simulink model "with_sssc"  (Simulink 7.3)
settings: Solver=FixedStepDiscrete  SolverMode=SingleTasking  StartTime=0.0  StopTime=0.8  FixedStep=Ts  RelTol=1e-3
PreLoadFcn:
  | Ts=1/512/60;
undefined symbols (not defined in the file): DiscIntNeverNeededParam
libraries: powerlib x54, powerlib_extras x38, simulink_extras x2, simulink x1
(part 3 of 7)

== system with_sssc/sssc Controller/SH Control (STATCOM)/DC Balance Regulator ==
  Iq_avg : Inport  PortDimensions=1  OutDataType=sfix(16)  OutScaling=2^0
  +/-Vdc/2 : Inport  Port=2  PortDimensions=2  OutDataType=sfix(16)  OutScaling=2^0
  " Mean value" : Subsystem  mask(Discrete Mean value){Freq=60, Vinit=0, Ts=Ts}
      mask prompts: Freq "Fundamental frequency (Hz):"; Vinit "Initial input (DC component):"; Ts "Sample time:"
      mask help:
      | This block computes the mean value of the input signal over a running window of one cycle of the specified fundamental frequency.
      | For the first cycle of simulation, the output is held constant to the value specified by the parameter "Initial input".
      mask init:
      | SamplesPerCycle=1/Freq/Ts;
      | RoundSamplesPerCycle=round(SamplesPerCycle);
      | Delay=RoundSamplesPerCycle*Ts - Ts/2;
      | Correction=SamplesPerCycle/RoundSamplesPerCycle - 1;
  Abs : Abs  OutDataType=sfix(16)  OutScaling=2^0  SaturateOnIntegerOverflow=on
  D_Alpha(Manual) : Constant  Value=0  OutDataType=sfix(16)  OutScaling=2^0
  D_Alpha1 : Constant  Value=0  OutDataType=sfix(16)  OutScaling=2^0
  D_Alpha2 : Constant  Value=0  OutDataType=sfix(16)  OutScaling=2^0
  D_Alpha5 : Constant  Value=0.1  OutDataType=sfix(16)  OutScaling=2^0
  Demux : Demux  Outputs=2
  Gain : Gain  Gain=0  ParameterDataType=sfix(16)  ParameterScaling=2^0  OutDataType=sfix(16)  OutScaling=2^0  SaturateOnIntegerOverflow=on  OutDataTypeStr=Inherit: Same as input  ParamDataTypeStr=Inherit: Same as input
  Gain1 : Gain  Gain=-1  ParameterDataType=sfix(16)  ParameterScaling=2^0  OutDataType=sfix(16)  OutScaling=2^0  SaturateOnIntegerOverflow=on  OutDataTypeStr=Inherit: Same as input  ParamDataTypeStr=Inherit: Same as input
  Mode : Constant  OutDataType=sfix(16)  OutScaling=2^0
  Multiport Switch : MultiPortSwitch  OutDataType=sfix(16)  OutScaling=2^0  SaturateOnIntegerOverflow=on  InputSameDT=on
  PI Regulator : Subsystem  mask(Discrete PI Controller){Kp=0.001, Ki=0.01, Par_Limits=[2 -2], Init=0, Ts=Ts}
      mask prompts: Kp "Proportional gain (Kp):"; Ki "Integral gain (Ki):"; Par_Limits "Output limits: [ Upper   Lower ]"; Init "Output initial value:"; Ts "Sample time:"
      mask help: This block implements a discrete PI controller.
      mask init:
      | UpperLimit=Par_Limits(1);
      | LowerLimit=Par_Limits(2);
      mask Display: disp('PI');
  Relational Operator : RelationalOperator  Operator=<=  InputSameDT=on
  Relational Operator1 : RelationalOperator  Operator=<  InputSameDT=on
  Sum2 : Sum  Inputs=-+  OutDataType=sfix(16)  OutScaling=2^0  SaturateOnIntegerOverflow=on  InputSameDT=on  OutDataTypeStr=Inherit: Same as first input
  Switch : Switch  Threshold=0.5  OutDataType=sfix(16)  OutScaling=2^0  SaturateOnIntegerOverflow=on  InputSameDT=on
  Switch1 : Switch  Threshold=0.5  OutDataType=sfix(16)  OutScaling=2^0  SaturateOnIntegerOverflow=on  InputSameDT=on
  D_Alpha : Outport  OutDataType=sfix(16)  OutScaling=2^0
  wires:
  Demux/2 -> Sum2/2
  Demux/1 -> Sum2/1
  +/-Vdc/2/1 -> Demux/1
  Iq_avg/1 -> Relational Operator/1, Abs/1
  Sum2/1 -> " Mean value"/1(In)
  Switch1/1 -> PI Regulator/1(Error)
  Gain/1 -> Switch1/1
  " Mean value"/1(Mean) -> Gain/1, Switch1/3
  D_Alpha1/1 -> Relational Operator/2
  Abs/1 -> Relational Operator1/1
  D_Alpha5/1 -> Relational Operator1/2
  Gain1/1 -> Switch/3
  Relational Operator/1 -> Switch/2
  Switch/1 -> Multiport Switch/2  "Auto"
  D_Alpha2/1 -> Multiport Switch/4  "Off"
  Mode/1 -> Multiport Switch/1
  PI Regulator/1(Out) -> Switch/1, Gain1/1
  D_Alpha(Manual)/1 -> Multiport Switch/3  "Man"
  Multiport Switch/1 -> D_Alpha/1
  Relational Operator1/1 -> Switch1/2, PI Regulator/2(Reset)

== system with_sssc/sssc Controller/SH Control (STATCOM)/Firing Pulses Generator ==
  Alpha : Inport  PortDimensions=1  OutDataType=sfix(16)  OutScaling=2^0
  Sigma : Inport  Port=2  PortDimensions=1  OutDataType=sfix(16)  OutScaling=2^0
  wt : Inport  Port=3  PortDimensions=1  OutDataType=sfix(16)  OutScaling=2^0
  D_Alpha : Inport  Port=4  PortDimensions=1  OutDataType=sfix(16)  OutScaling=2^0
  " Deg->Rad" : Gain  Gain=pi/180  ParameterDataType=sfix(16)  ParameterScaling=2^0  OutDataType=sfix(16)  OutScaling=2^0  SaturateOnIntegerOverflow=on  OutDataTypeStr=Inherit: Same as input  ParamDataTypeStr=Inherit: Same as input
  Bridge 1D : Subsystem
  "Bridge 1Y " : Subsystem
  Bridge 2D : Subsystem
  Bridge 2Y : Subsystem
  Constant : Constant  Value=[0 -30 -15 -45]*pi/180 + 7.5*pi/180  OutDataType=sfix(16)  OutScaling=2^0
  Deg->Rad : Gain  Gain=pi/180  ParameterDataType=sfix(16)  ParameterScaling=2^0  OutDataType=sfix(16)  OutScaling=2^0  SaturateOnIntegerOverflow=on  OutDataTypeStr=Inherit: Same as input  ParamDataTypeStr=Inherit: Same as input
  "Deg->Rad " : Gain  Gain=pi/180  ParameterDataType=sfix(16)  ParameterScaling=2^0  OutDataType=sfix(16)  OutScaling=2^0  SaturateOnIntegerOverflow=on  OutDataTypeStr=Inherit: Same as input  ParamDataTypeStr=Inherit: Same as input
  Demux : Demux
  Mux : Mux  Inputs=[12 12 12 12]
  Sum : Sum  OutDataType=sfix(16)  OutScaling=2^0  SaturateOnIntegerOverflow=on  InputSameDT=on  OutDataTypeStr=Inherit: Same as first input
  Pulses : Outport  OutDataType=sfix(16)  OutScaling=2^0
  wires:
  Alpha/1 -> Deg->Rad/1
  Constant/1 -> Sum/2
  Sum/1 -> Demux/1
  "Bridge 1Y "/1(Pulses) -> Mux/1
  Mux/1 -> Pulses/1
  Demux/1 -> "Bridge 1Y "/1(wt)
  Sigma/1 -> "Deg->Rad "/1
  Demux/2 -> Bridge 1D/1(wt)
  Demux/3 -> Bridge 2Y/1(wt)
  Demux/4 -> Bridge 2D/1(wt)
  Deg->Rad/1 -> "Bridge 1Y "/2(Alpha), Bridge 1D/2(Alpha), Bridge 2Y/2(Alpha), Bridge 2D/2(Alpha)
  "Deg->Rad "/1 -> "Bridge 1Y "/3(Sigma), Bridge 1D/3(Sigma), Bridge 2Y/3(Sigma), Bridge 2D/3(Sigma)
  " Deg->Rad"/1 -> Bridge 2D/4(D_Alpha), Bridge 2Y/4(D_Alpha), Bridge 1D/4(D_Alpha), "Bridge 1Y "/4(D_Alpha)
  D_Alpha/1 -> " Deg->Rad"/1
  Bridge 1D/1(Pulses) -> Mux/2
  Bridge 2Y/1(Pulses) -> Mux/3
  Bridge 2D/1(Pulses) -> Mux/4
  wt/1 -> Sum/1

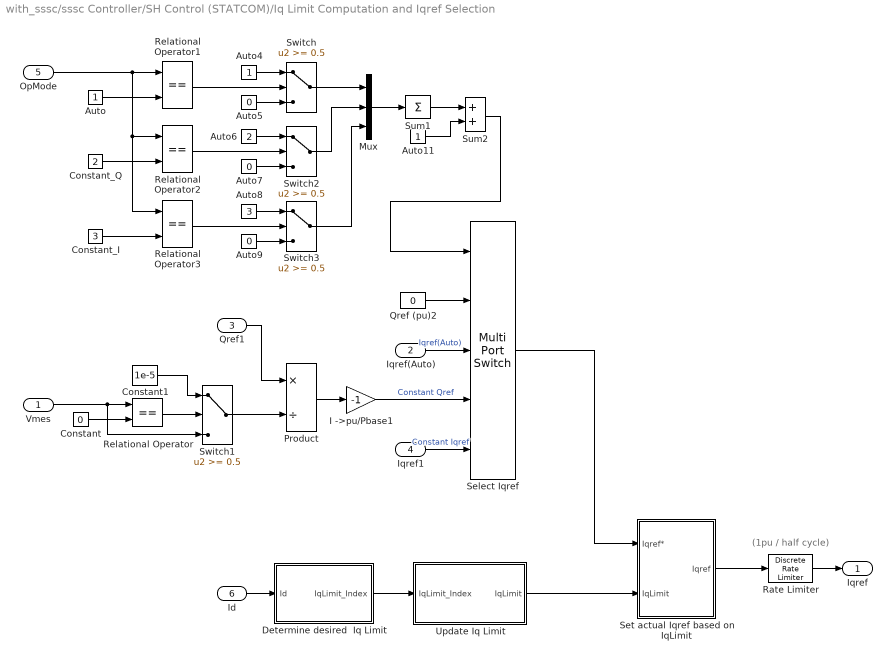
== system with_sssc/sssc Controller/SH Control (STATCOM)/Iq Limit Computation and Iqref Selection ==
  note: (1pu / half cycle)
  Vmes : Inport  OutDataType=sfix(16)  OutScaling=2^0
  Iqref(Auto) : Inport  Port=2  OutDataType=sfix(16)  OutScaling=2^0
  Qref1 : Inport  Port=3  OutDataType=sfix(16)  OutScaling=2^0
  Iqref1 : Inport  Port=4  OutDataType=sfix(16)  OutScaling=2^0
  OpMode : Inport  Port=5  OutDataType=sfix(16)  OutScaling=2^0
  Id : Inport  Port=6  OutDataType=sfix(16)  OutScaling=2^0
  Auto : Constant  OutDataType=sfix(16)  OutScaling=2^0
  Auto11 : Constant  OutDataType=sfix(16)  OutScaling=2^0
  Auto4 : Constant  OutDataType=sfix(16)  OutScaling=2^0
  Auto5 : Constant  Value=0  OutDataType=sfix(16)  OutScaling=2^0
  Auto6 : Constant  Value=2  OutDataType=sfix(16)  OutScaling=2^0
  Auto7 : Constant  Value=0  OutDataType=sfix(16)  OutScaling=2^0
  Auto8 : Constant  Value=3  OutDataType=sfix(16)  OutScaling=2^0
  Auto9 : Constant  Value=0  OutDataType=sfix(16)  OutScaling=2^0
  Constant : Constant  Value=0  OutDataType=sfix(16)  OutScaling=2^0
  Constant1 : Constant  Value=1e-5  OutDataType=sfix(16)  OutScaling=2^0
  Constant_I : Constant  Value=3  OutDataType=sfix(16)  OutScaling=2^0
  Constant_Q : Constant  Value=2  OutDataType=sfix(16)  OutScaling=2^0
  Determine desired  Iq Limit : Subsystem
  I ->pu/Pbase1 : Gain  Gain=-1  ParameterDataType=sfix(16)  ParameterScaling=2^0  OutDataType=sfix(16)  OutScaling=2^0  SaturateOnIntegerOverflow=on  OutDataTypeStr=Inherit: Same as input  ParamDataTypeStr=Inherit: Same as input
  Mux : Mux  Inputs=3
  Product : Product  Inputs=*/  OutDataType=sfix(16)  OutScaling=2^0  SaturateOnIntegerOverflow=on  InputSameDT=on  OutDataTypeStr=Inherit: Same as first input
  Qref (pu)2 : Constant  Value=0  OutDataType=sfix(16)  OutScaling=2^0
  "Rate Limiter " : powerlib_extras/Discrete  Control Blocks/Discrete Rate Limiter  DialogController=POWERSYS.PowerSysDialog  SystemSampleTime=-1  R=120  F=-120  Vinit=-0.33  Ts=Ts
  Relational Operator{,1..3} (4 alike) : RelationalOperator  Operator===  InputSameDT=on
  Select Iqref : MultiPortSwitch  Inputs=4  OutDataType=sfix(16)  OutScaling=2^0  SaturateOnIntegerOverflow=on  InputSameDT=on
  Set actual Iqref based on IqLimit : Subsystem
  Sum1 : Sum  Inputs=1  OutDataType=sfix(16)  OutScaling=2^0  SaturateOnIntegerOverflow=on  InputSameDT=on  OutDataTypeStr=Inherit: Same as first input
  Sum2 : Sum  OutDataType=sfix(16)  OutScaling=2^0  SaturateOnIntegerOverflow=on  InputSameDT=on  OutDataTypeStr=Inherit: Same as first input
  Switch{,1..3} (4 alike) : Switch  Threshold=0.5  OutDataType=sfix(16)  OutScaling=2^0  SaturateOnIntegerOverflow=on  InputSameDT=on
  Update Iq Limit : Subsystem
  Iqref : Outport  OutDataType=sfix(16)  OutScaling=2^0
  wires:
  Switch2/1 -> Mux/2
  Auto11/1 -> Sum2/2
  Sum1/1 -> Sum2/1
  Switch3/1 -> Mux/3
  Mux/1 -> Sum1/1
  Switch/1 -> Mux/1
  Auto9/1 -> Switch3/3
  Auto8/1 -> Switch3/1
  Relational Operator3/1 -> Switch3/2
  Auto7/1 -> Switch2/3
  Auto6/1 -> Switch2/1
  Relational Operator2/1 -> Switch2/2
  Auto5/1 -> Switch/3
  Auto4/1 -> Switch/1
  Relational Operator1/1 -> Switch/2
  OpMode/1 -> Relational Operator3/1, Relational Operator2/1, Relational Operator1/1
  Constant_I/1 -> Relational Operator3/2
  Constant_Q/1 -> Relational Operator2/2
  Auto/1 -> Relational Operator1/2
  Sum2/1 -> Select Iqref/1
  Vmes/1 -> Relational Operator/1, Switch1/3
  Qref1/1 -> Product/1
  Relational Operator/1 -> Switch1/2
  Constant1/1 -> Switch1/1
  Switch1/1 -> Product/2
  Constant/1 -> Relational Operator/2
  Product/1 -> I ->pu/Pbase1/1
  Iqref1/1 -> Select Iqref/5  "Constant Iqref"
  Iqref(Auto)/1 -> Select Iqref/3  "Iqref(Auto)"
  I ->pu/Pbase1/1 -> Select Iqref/4  "Constant Qref"
  Qref (pu)2/1 -> Select Iqref/2
  Select Iqref/1 -> Set actual Iqref based on IqLimit/1(Iqref*)
  Determine desired  Iq Limit/1(IqLimit_Index) -> Update Iq Limit/1(IqLimit_Index)
  Update Iq Limit/1(IqLimit) -> Set actual Iqref based on IqLimit/2(IqLimit)
  Set actual Iqref based on IqLimit/1(Iqref) -> "Rate Limiter "/1
  "Rate Limiter "/1 -> Iqref/1
  Id/1 -> Determine desired  Iq Limit/1(Id)

== system with_sssc/sssc Controller/SH Control (STATCOM)/Measurement System ==
  Vabc : Inport  PortDimensions=3  OutDataType=sfix(16)  OutScaling=2^0
  Iabc : Inport  Port=2  PortDimensions=3  OutDataType=sfix(16)  OutScaling=2^0
  Freq : Inport  Port=3  PortDimensions=1  OutDataType=sfix(16)  OutScaling=2^0
  wt : Inport  Port=4  PortDimensions=1  OutDataType=sfix(16)  OutScaling=2^0
  Discrete Variable Frequency Mean value : powerlib_extras/Discrete Measurements/Discrete Variable Frequency Mean value  DialogController=POWERSYS.PowerSysDialog  SystemSampleTime=-1  Finit=60  Fmin=45  Vinit=0  Ts=Ts
  Discrete  2nd-Order Filter : powerlib_extras/Discrete  Control Blocks/Discrete  2nd-Order Filter  DialogController=POWERSYS.PowerSysDialog  SystemSampleTime=-1  FilterType=Lowpass  Fo=1200  Zeta=0.707  Ts=Ts  Initialize=off  Vac_Init=[0.8 -25 60]  Vdc_Init=-0.4  PlotResponse=off  param1=[1 500 1]
  Discrete  2nd-Order Filter1 : powerlib_extras/Discrete  Control Blocks/Discrete  2nd-Order Filter  DialogController=POWERSYS.PowerSysDialog  SystemSampleTime=-1  FilterType=Lowpass  Fo=1200  Zeta=0.707  Ts=Ts  Initialize=off  Vac_Init=[0.8 -25 60]  Vdc_Init=-0.4  PlotResponse=off  param1=[1 500 1]
  Mux : Mux  Inputs=2
  PQ  Computaion : Subsystem
  Selector : Selector  InputPortWidth=2  IndexOptions=Index vector (dialog)  Indices=2  OutputSizes=1
  Selector1 : Selector  InputPortWidth=2  IndexOptions=Index vector (dialog)  Indices=1  OutputSizes=1
  Selector2 : Selector  InputPortWidth=3  IndexOptions=Index vector (dialog)  Indices=1:2  OutputSizes=1
  Trigonometric Function : Trigonometry
  Trigonometric Function1 : Trigonometry  Operator=cos
  Voltage measurement (Positive sequence) : Subsystem  mask(Discrete 3-phase PLL-Driven Positive-Sequence Fundamental Value){Finit=60, Par_Init=[1 0], Ts=Ts}
      mask prompts: Finit "Initial fundamental frequency (Hz):"; Par_Init "Initial input (positive component): [ Mag  Phase-relative-to-PLL(degrees) ]"; Ts "Sample time:"
      mask help:
      | For a supplied fundamental frequency (port Freq), this discrete block computes  the positive-sequence component (Magnitude and Phase)  of a set of three balanced or unbalanced signals (port abc) which may contain harmonics.
      |  Input port "Sin_Cos" (a two-dimension signal) provides the reference frame required for the computation..
      |  First and second outputs return respectively the magnitude and phase (in degrees relative to the PLL phase)) of the fundamental.
      | For the first cycle of simulation, the outputs are held constant to the values specified by the parameter "Initial input".
      mask init:
      | Real_Init=Par_Init(1)*cos(pi/180*Par_Init(2));
      | Imag_Init=Par_Init(1)*sin(pi/180*Par_Init(2));
  abc_to_dq0 Transformation : powerlib_extras/Measurements/abc_to_dq0 Transformation  DialogController=POWERSYS.PowerSysDialog  SystemSampleTime=-1
  Vmes : Outport  OutDataType=sfix(16)  OutScaling=2^0
  PQ : Outport  Port=2  OutDataType=sfix(16)  OutScaling=2^0
  Iq : Outport  Port=3  OutDataType=sfix(16)  OutScaling=2^0
  Iq_avg : Outport  Port=4  OutDataType=sfix(16)  OutScaling=2^0
  Id : Outport  Port=5  OutDataType=sfix(16)  OutScaling=2^0
  wires:
  Discrete  2nd-Order Filter/1 -> Id/1
  Selector1/1 -> Discrete  2nd-Order Filter/1
  Discrete Variable Frequency Mean value/1 -> Iq_avg/1
  Selector/1 -> Discrete  2nd-Order Filter1/1, Discrete Variable Frequency Mean value/2
  Freq/1 -> PQ  Computaion/3(Freq), Discrete Variable Frequency Mean value/1, Voltage measurement (Positive sequence)/2(Freq)
  abc_to_dq0 Transformation/1 -> Selector2/1
  PQ  Computaion/1(PQ(pu)) -> PQ/1
  Mux/1 -> Voltage measurement (Positive sequence)/3(Sin_Cos), abc_to_dq0 Transformation/2
  wt/1 -> Trigonometric Function1/1, Trigonometric Function/1
  Trigonometric Function1/1 -> Mux/2
  Trigonometric Function/1 -> Mux/1
  Vabc/1 -> Voltage measurement (Positive sequence)/1(abc)
  Voltage measurement (Positive sequence)/1(Mag) -> Vmes/1  "Vmes"
  Voltage measurement (Positive sequence)/2(VdVq) -> PQ  Computaion/1(Vd_Vq)
  Discrete  2nd-Order Filter1/1 -> Iq/1
  Iabc/1 -> abc_to_dq0 Transformation/1
  Selector2/1 -> Selector1/1, Selector/1, PQ  Computaion/2(Id_Iq)

== system with_sssc/sssc Controller/SH Control (STATCOM)/PLL ==
  note: Pierre Giroux, Gilbert Sybille
      | Power System Laboratory, IREQ
      | Hydro-Quebec
  note: Discrete 3-phase PLL
  Vabc (pu) : Inport  PortDimensions=3  OutDataType=sfix(16)  OutScaling=2^0
  Constant4 : Constant  Value=2*pi  OutDataType=sfix(16)  OutScaling=2^0
  Correction for delay : Gain  Gain=Nstep*Ts*2*pi  ParameterDataType=sfix(16)  ParameterScaling=2^0  OutDataType=sfix(16)  OutScaling=2^0  SaturateOnIntegerOverflow=on  OutDataTypeStr=Inherit: Same as input  ParamDataTypeStr=Inherit: Same as input
  Discrete PI Controller : powerlib_extras/Discrete  Control Blocks/Discrete PI Controller  DialogController=POWERSYS.PowerSysDialog  SystemSampleTime=-1  Kp=Kp  Ki=Ki  Par_Limits=2*pi*Finit*[1.25 0.75]  Init=2*pi*Finit  Ts=Ts
  Discrete Rate Limiter : powerlib_extras/Discrete  Control Blocks/Discrete Rate Limiter  DialogController=POWERSYS.PowerSysDialog  SystemSampleTime=-1  R=10  F=-10  Vinit=Finit  Ts=Ts
  Discrete Variable Frequency Mean value : Subsystem  mask(Discrete Variable-Frequency Mean Value){Finit=Finit, Vinit=0, Ts=Ts}
      mask prompts: Finit "Initial Frequency (Hz):"; Vinit "Initial input (DC component):"; Ts "Sample time:"
      mask help:
      | This discrete block computes the mean value of the input signal (port In) over a running window of one cycle of a specified frequency (port Freq).
      |
      | For the first cycle of simulation (specified by the parameter "Initial frequency"), the output is held to the value of the  "Initial input" parameter.
  Discrete  2nd-Order Filter : powerlib_extras/Discrete  Control Blocks/Discrete  2nd-Order Filter  DialogController=POWERSYS.PowerSysDialog  SystemSampleTime=-1  FilterType=Lowpass  Fo=25  Zeta=0.707  Ts=Ts  Initialize=on  Vac_Init=[0 -25 60]  Vdc_Init=Finit  PlotResponse=off  param1=[1 500 0.1]
  Discrete-Time Integrator : DiscreteIntegrator  InitialCondition=Phase_Init*pi/180  SampleTime=Ts  OutDataType=sfix(16)  OutScaling=2^0  ICPrevOutput=DiscIntNeverNeededParam  ICPrevScaledInput=DiscIntNeverNeededParam
  Gain10 : Gain  Gain=1/2/pi  ParameterDataType=sfix(16)  ParameterScaling=2^0  OutDataType=sfix(16)  OutScaling=2^0  SaturateOnIntegerOverflow=on  OutDataTypeStr=Inherit: Same as input  ParamDataTypeStr=Inherit: Same as input
  Math Function : Math  Operator=mod  OutDataType=sfix(16)  OutScaling=2^0  SaturateOnIntegerOverflow=on
  Mux2 : Mux  Inputs=2
  Selector : Selector  InputPortWidth=3  IndexOptions=Index vector (dialog)  Indices=2  OutputSizes=1
  Sum : Sum  OutDataType=sfix(16)  OutScaling=2^0  SaturateOnIntegerOverflow=on  InputSameDT=on  OutDataTypeStr=Inherit: Same as first input
  Trigonometric Function : Trigonometry
  Trigonometric Function2 : Trigonometry  Operator=cos
  Unit Delay : UnitDelay  X0=Finit  SampleTime=Ts
  abc_to_dq0 Transformation : powerlib_extras/Measurements/abc_to_dq0 Transformation  DialogController=POWERSYS.PowerSysDialog  SystemSampleTime=-1
  Freq : Outport  OutDataType=sfix(16)  OutScaling=2^0
  wt : Outport  Port=2  OutDataType=sfix(16)  OutScaling=2^0
  wires:
  Sum/1 -> wt/1
  Selector/1 -> Discrete Variable Frequency Mean value/2(In)  "Vq"
  Discrete  2nd-Order Filter/1 -> Unit Delay/1
  Unit Delay/1 -> Freq/1, Discrete Variable Frequency Mean value/1(Freq), Correction for delay/1
  Discrete Rate Limiter/1 -> Discrete  2nd-Order Filter/1
  Gain10/1 -> Discrete Rate Limiter/1
  Discrete PI Controller/1 -> Gain10/1, Discrete-Time Integrator/1  "W"
  Trigonometric Function2/1 -> Mux2/2
  Trigonometric Function/1 -> Mux2/1
  Math Function/1 -> Trigonometric Function2/1, Trigonometric Function/1, Sum/2
  Discrete-Time Integrator/1 -> Math Function/1
  Constant4/1 -> Math Function/2
  abc_to_dq0 Transformation/1 -> Selector/1
  Vabc (pu)/1 -> abc_to_dq0 Transformation/1
  Discrete Variable Frequency Mean value/1(Mean) -> Discrete PI Controller/1
  Mux2/1 -> abc_to_dq0 Transformation/2
  Correction for delay/1 -> Sum/1

== system with_sssc/sssc Controller/SH Control (STATCOM)/Voltage  Regulator ==
  Vref : Inport  OutDataType=sfix(16)  OutScaling=2^0
  Vmes : Inport  Port=2  OutDataType=sfix(16)  OutScaling=2^0
  Discrete-Time Integrator : DiscreteIntegrator  InitialCondition=Init  SampleTime=Ts  OutDataType=sfix(16)  OutScaling=2^0  LimitOutput=on  UpperSaturationLimit=UpperLimit  LowerSaturationLimit=LowerLimit  ICPrevOutput=DiscIntNeverNeededParam  ICPrevScaledInput=DiscIntNeverNeededParam
  Kp4 : Gain  Gain=Kp  ParameterDataType=sfix(16)  ParameterScaling=2^0  OutDataType=sfix(16)  OutScaling=2^0  SaturateOnIntegerOverflow=on  OutDataTypeStr=Inherit: Same as input  ParamDataTypeStr=Inherit: Same as input
  Kp5 : Gain  Gain=Ki  ParameterDataType=sfix(16)  ParameterScaling=2^0  OutDataType=sfix(16)  OutScaling=2^0  SaturateOnIntegerOverflow=on  OutDataTypeStr=Inherit: Same as input  ParamDataTypeStr=Inherit: Same as input
  Kp6 : Gain  Gain=Droop  ParameterDataType=sfix(16)  ParameterScaling=2^0  OutDataType=sfix(16)  OutScaling=2^0  SaturateOnIntegerOverflow=on  OutDataTypeStr=Inherit: Same as input  ParamDataTypeStr=Inherit: Same as input
  Saturation2 : Saturate  UpperLimit=UpperLimit  LowerLimit=LowerLimit  OutDataType=sfix(16)  OutScaling=2^0
  Sum1 : Sum  Inputs=|-+  OutDataType=sfix(16)  OutScaling=2^0  SaturateOnIntegerOverflow=on  InputSameDT=on  OutDataTypeStr=Inherit: Same as first input
  Sum6 : Sum  OutDataType=sfix(16)  OutScaling=2^0  SaturateOnIntegerOverflow=on  InputSameDT=on  OutDataTypeStr=Inherit: Same as first input
  Sum7 : Sum  Inputs=|+-  OutDataType=sfix(16)  OutScaling=2^0  SaturateOnIntegerOverflow=on  InputSameDT=on  OutDataTypeStr=Inherit: Same as first input
  Unit Delay : UnitDelay  SampleTime=Ts
  Iqref : Outport  OutDataType=sfix(16)  OutScaling=2^0  InitialOutput=0
  wires:
  Sum1/1 -> Sum7/1  "Err"
  Vref/1 -> Sum1/2
  Vmes/1 -> Sum1/1
  Unit Delay/1 -> Sum7/2
  Kp6/1 -> Unit Delay/1
  Saturation2/1 -> Kp6/1, Iqref/1  "Iq_Ref"
  Sum7/1 -> Kp4/1, Kp5/1
  Kp5/1 -> Discrete-Time Integrator/1
  Sum6/1 -> Saturation2/1
  Kp4/1 -> Sum6/1
  Discrete-Time Integrator/1 -> Sum6/2

== system with_sssc/sssc Controller/SE Control (SSSC)/Firing Pulses Generator/Bridge 1D ==
  wt : Inport  PortDimensions=1  OutDataType=sfix(16)  OutScaling=2^0
  Alpha : Inport  Port=2  PortDimensions=1  OutDataType=sfix(16)  OutScaling=2^0
  Sigma : Inport  Port=3  PortDimensions=1  OutDataType=sfix(16)  OutScaling=2^0
  D_Alpha : Inport  Port=4  PortDimensions=1  OutDataType=sfix(16)  OutScaling=2^0
  Constant : Constant  Value=-2*pi/3  OutDataType=sfix(16)  OutScaling=2^0
  Constant1 : Constant  Value=2*pi/3  OutDataType=sfix(16)  OutScaling=2^0
  Mux1 : Mux  Inputs=[4 4 4]
  Phase A : Subsystem
  Phase B : Subsystem
  Phase C : Subsystem
  Sum : Sum  OutDataType=sfix(16)  OutScaling=2^0  SaturateOnIntegerOverflow=on  InputSameDT=on  OutDataTypeStr=Inherit: Same as first input
  Sum1 : Sum  OutDataType=sfix(16)  OutScaling=2^0  SaturateOnIntegerOverflow=on  InputSameDT=on  OutDataTypeStr=Inherit: Same as first input
  Sum2 : Sum  OutDataType=sfix(16)  OutScaling=2^0  SaturateOnIntegerOverflow=on  InputSameDT=on  OutDataTypeStr=Inherit: Same as first input
  Pulses : Outport  OutDataType=sfix(16)  OutScaling=2^0
  wires:
  Constant1/1 -> Sum1/2
  Sigma/1 -> Phase A/2(sigma), Phase C/2(sigma), Phase B/2(sigma)
  Alpha/1 -> Sum2/2
  wt/1 -> Sum2/1
  Sum2/1 -> Phase A/1(wt), Sum/1, Sum1/1
  Mux1/1 -> Pulses/1
  Phase A/1(Pulses) -> Mux1/1
  Constant/1 -> Sum/2
  Sum/1 -> Phase B/1(wt)
  Sum1/1 -> Phase C/1(wt)
  D_Alpha/1 -> Phase A/3(D_Alpha), Phase B/3(D_Alpha), Phase C/3(D_Alpha)
  Phase B/1(Pulses) -> Mux1/2
  Phase C/1(Pulses) -> Mux1/3

== system with_sssc/sssc Controller/SE Control (SSSC)/Firing Pulses Generator/Bridge 1Y  ==
  wt : Inport  PortDimensions=1  OutDataType=sfix(16)  OutScaling=2^0
  Alpha : Inport  Port=2  PortDimensions=1  OutDataType=sfix(16)  OutScaling=2^0
  Sigma : Inport  Port=3  PortDimensions=1  OutDataType=sfix(16)  OutScaling=2^0
  D_Alpha : Inport  Port=4  PortDimensions=1  OutDataType=sfix(16)  OutScaling=2^0
  Constant : Constant  Value=-2*pi/3  OutDataType=sfix(16)  OutScaling=2^0
  Constant1 : Constant  Value=2*pi/3  OutDataType=sfix(16)  OutScaling=2^0
  Mux1 : Mux  Inputs=[4 4 4]
  Phase A : Subsystem
  Phase B : Subsystem
  Phase C : Subsystem
  Sum : Sum  OutDataType=sfix(16)  OutScaling=2^0  SaturateOnIntegerOverflow=on  InputSameDT=on  OutDataTypeStr=Inherit: Same as first input
  Sum1 : Sum  OutDataType=sfix(16)  OutScaling=2^0  SaturateOnIntegerOverflow=on  InputSameDT=on  OutDataTypeStr=Inherit: Same as first input
  Sum2 : Sum  OutDataType=sfix(16)  OutScaling=2^0  SaturateOnIntegerOverflow=on  InputSameDT=on  OutDataTypeStr=Inherit: Same as first input
  Pulses : Outport  OutDataType=sfix(16)  OutScaling=2^0
  wires:
  Phase C/1(Pulses) -> Mux1/3
  Phase B/1(Pulses) -> Mux1/2
  D_Alpha/1 -> Phase C/3(D_Alpha), Phase B/3(D_Alpha), Phase A/3(D_Alpha)
  Sum1/1 -> Phase C/1(wt)
  Sum/1 -> Phase B/1(wt)
  Constant/1 -> Sum/2
  Phase A/1(Pulses) -> Mux1/1
  Mux1/1 -> Pulses/1
  Sum2/1 -> Sum1/1, Sum/1, Phase A/1(wt)
  wt/1 -> Sum2/1
  Alpha/1 -> Sum2/2
  Sigma/1 -> Phase B/2(sigma), Phase C/2(sigma), Phase A/2(sigma)
  Constant1/1 -> Sum1/2

== system with_sssc/sssc Controller/SE Control (SSSC)/Firing Pulses Generator/Bridge 2D ==
  wt : Inport  PortDimensions=1  OutDataType=sfix(16)  OutScaling=2^0
  Alpha : Inport  Port=2  PortDimensions=1  OutDataType=sfix(16)  OutScaling=2^0
  Sigma : Inport  Port=3  PortDimensions=1  OutDataType=sfix(16)  OutScaling=2^0
  D_Alpha : Inport  Port=4  PortDimensions=1  OutDataType=sfix(16)  OutScaling=2^0
  Constant : Constant  Value=-2*pi/3  OutDataType=sfix(16)  OutScaling=2^0
  Constant1 : Constant  Value=2*pi/3  OutDataType=sfix(16)  OutScaling=2^0
  Mux1 : Mux  Inputs=[4 4 4]
  Phase A : Subsystem
  Phase B : Subsystem
  Phase C : Subsystem
  Sum : Sum  OutDataType=sfix(16)  OutScaling=2^0  SaturateOnIntegerOverflow=on  InputSameDT=on  OutDataTypeStr=Inherit: Same as first input
  Sum1 : Sum  OutDataType=sfix(16)  OutScaling=2^0  SaturateOnIntegerOverflow=on  InputSameDT=on  OutDataTypeStr=Inherit: Same as first input
  Sum2 : Sum  OutDataType=sfix(16)  OutScaling=2^0  SaturateOnIntegerOverflow=on  InputSameDT=on  OutDataTypeStr=Inherit: Same as first input
  Pulses : Outport  OutDataType=sfix(16)  OutScaling=2^0
  wires:
  Constant1/1 -> Sum1/2
  Sigma/1 -> Phase A/2(sigma), Phase C/2(sigma), Phase B/2(sigma)
  Alpha/1 -> Sum2/2
  wt/1 -> Sum2/1
  Sum2/1 -> Phase A/1(wt), Sum/1, Sum1/1
  Mux1/1 -> Pulses/1
  Phase A/1(Pulses) -> Mux1/1
  Constant/1 -> Sum/2
  Sum/1 -> Phase B/1(wt)
  Sum1/1 -> Phase C/1(wt)
  D_Alpha/1 -> Phase A/3(D_Alpha), Phase B/3(D_Alpha), Phase C/3(D_Alpha)
  Phase B/1(Pulses) -> Mux1/2
  Phase C/1(Pulses) -> Mux1/3

== system with_sssc/sssc Controller/SE Control (SSSC)/Firing Pulses Generator/Bridge 2Y ==
  wt : Inport  PortDimensions=1  OutDataType=sfix(16)  OutScaling=2^0
  Alpha : Inport  Port=2  PortDimensions=1  OutDataType=sfix(16)  OutScaling=2^0
  Sigma : Inport  Port=3  PortDimensions=1  OutDataType=sfix(16)  OutScaling=2^0
  D_Alpha : Inport  Port=4  PortDimensions=1  OutDataType=sfix(16)  OutScaling=2^0
  Constant : Constant  Value=-2*pi/3  OutDataType=sfix(16)  OutScaling=2^0
  Constant1 : Constant  Value=2*pi/3  OutDataType=sfix(16)  OutScaling=2^0
  Mux1 : Mux  Inputs=[4 4 4]
  Phase A : Subsystem
  Phase B : Subsystem
  Phase C : Subsystem
  Sum : Sum  OutDataType=sfix(16)  OutScaling=2^0  SaturateOnIntegerOverflow=on  InputSameDT=on  OutDataTypeStr=Inherit: Same as first input
  Sum1 : Sum  OutDataType=sfix(16)  OutScaling=2^0  SaturateOnIntegerOverflow=on  InputSameDT=on  OutDataTypeStr=Inherit: Same as first input
  Sum2 : Sum  OutDataType=sfix(16)  OutScaling=2^0  SaturateOnIntegerOverflow=on  InputSameDT=on  OutDataTypeStr=Inherit: Same as first input
  Pulses : Outport  OutDataType=sfix(16)  OutScaling=2^0
  wires:
  Phase C/1(Pulses) -> Mux1/3
  Phase B/1(Pulses) -> Mux1/2
  D_Alpha/1 -> Phase C/3(D_Alpha), Phase B/3(D_Alpha), Phase A/3(D_Alpha)
  Sum1/1 -> Phase C/1(wt)
  Sum/1 -> Phase B/1(wt)
  Constant/1 -> Sum/2
  Phase A/1(Pulses) -> Mux1/1
  Mux1/1 -> Pulses/1
  Sum2/1 -> Sum1/1, Sum/1, Phase A/1(wt)
  wt/1 -> Sum2/1
  Alpha/1 -> Sum2/2
  Sigma/1 -> Phase B/2(sigma), Phase C/2(sigma), Phase A/2(sigma)
  Constant1/1 -> Sum1/2

== system with_sssc/sssc Controller/SE Control (UPFC)/Firing Pulses Generator/Bridge 1D ==
  wt : Inport  PortDimensions=1  OutDataType=sfix(16)  OutScaling=2^0
  Alpha : Inport  Port=2  PortDimensions=1  OutDataType=sfix(16)  OutScaling=2^0
  Sigma : Inport  Port=3  PortDimensions=1  OutDataType=sfix(16)  OutScaling=2^0
  D_Alpha : Inport  Port=4  PortDimensions=1  OutDataType=sfix(16)  OutScaling=2^0
  Constant : Constant  Value=-2*pi/3  OutDataType=sfix(16)  OutScaling=2^0
  Constant1 : Constant  Value=2*pi/3  OutDataType=sfix(16)  OutScaling=2^0
  Mux1 : Mux  Inputs=[4 4 4]
  Phase A : Subsystem
  Phase B : Subsystem
  Phase C : Subsystem
  Sum : Sum  OutDataType=sfix(16)  OutScaling=2^0  SaturateOnIntegerOverflow=on  InputSameDT=on  OutDataTypeStr=Inherit: Same as first input
  Sum1 : Sum  OutDataType=sfix(16)  OutScaling=2^0  SaturateOnIntegerOverflow=on  InputSameDT=on  OutDataTypeStr=Inherit: Same as first input
  Sum2 : Sum  OutDataType=sfix(16)  OutScaling=2^0  SaturateOnIntegerOverflow=on  InputSameDT=on  OutDataTypeStr=Inherit: Same as first input
  Pulses : Outport  OutDataType=sfix(16)  OutScaling=2^0
  wires:
  Constant1/1 -> Sum1/2
  Sigma/1 -> Phase A/2(sigma), Phase C/2(sigma), Phase B/2(sigma)
  Alpha/1 -> Sum2/2
  wt/1 -> Sum2/1
  Sum2/1 -> Phase A/1(wt), Sum/1, Sum1/1
  Mux1/1 -> Pulses/1
  Phase A/1(Pulses) -> Mux1/1
  Constant/1 -> Sum/2
  Sum/1 -> Phase B/1(wt)
  Sum1/1 -> Phase C/1(wt)
  D_Alpha/1 -> Phase A/3(D_Alpha), Phase B/3(D_Alpha), Phase C/3(D_Alpha)
  Phase B/1(Pulses) -> Mux1/2
  Phase C/1(Pulses) -> Mux1/3

== system with_sssc/sssc Controller/SE Control (UPFC)/Firing Pulses Generator/Bridge 1Y  ==
  wt : Inport  PortDimensions=1  OutDataType=sfix(16)  OutScaling=2^0
  Alpha : Inport  Port=2  PortDimensions=1  OutDataType=sfix(16)  OutScaling=2^0
  Sigma : Inport  Port=3  PortDimensions=1  OutDataType=sfix(16)  OutScaling=2^0
  D_Alpha : Inport  Port=4  PortDimensions=1  OutDataType=sfix(16)  OutScaling=2^0
  Constant : Constant  Value=-2*pi/3  OutDataType=sfix(16)  OutScaling=2^0
  Constant1 : Constant  Value=2*pi/3  OutDataType=sfix(16)  OutScaling=2^0
  Mux1 : Mux  Inputs=[4 4 4]
  Phase A : Subsystem
  Phase B : Subsystem
  Phase C : Subsystem
  Sum : Sum  OutDataType=sfix(16)  OutScaling=2^0  SaturateOnIntegerOverflow=on  InputSameDT=on  OutDataTypeStr=Inherit: Same as first input
  Sum1 : Sum  OutDataType=sfix(16)  OutScaling=2^0  SaturateOnIntegerOverflow=on  InputSameDT=on  OutDataTypeStr=Inherit: Same as first input
  Sum2 : Sum  OutDataType=sfix(16)  OutScaling=2^0  SaturateOnIntegerOverflow=on  InputSameDT=on  OutDataTypeStr=Inherit: Same as first input
  Pulses : Outport  OutDataType=sfix(16)  OutScaling=2^0
  wires:
  Phase C/1(Pulses) -> Mux1/3
  Phase B/1(Pulses) -> Mux1/2
  D_Alpha/1 -> Phase C/3(D_Alpha), Phase B/3(D_Alpha), Phase A/3(D_Alpha)
  Sum1/1 -> Phase C/1(wt)
  Sum/1 -> Phase B/1(wt)
  Constant/1 -> Sum/2
  Phase A/1(Pulses) -> Mux1/1
  Mux1/1 -> Pulses/1
  Sum2/1 -> Sum1/1, Sum/1, Phase A/1(wt)
  wt/1 -> Sum2/1
  Alpha/1 -> Sum2/2
  Sigma/1 -> Phase B/2(sigma), Phase C/2(sigma), Phase A/2(sigma)
  Constant1/1 -> Sum1/2

== system with_sssc/sssc Controller/SE Control (UPFC)/Firing Pulses Generator/Bridge 2D ==
  wt : Inport  PortDimensions=1  OutDataType=sfix(16)  OutScaling=2^0
  Alpha : Inport  Port=2  PortDimensions=1  OutDataType=sfix(16)  OutScaling=2^0
  Sigma : Inport  Port=3  PortDimensions=1  OutDataType=sfix(16)  OutScaling=2^0
  D_Alpha : Inport  Port=4  PortDimensions=1  OutDataType=sfix(16)  OutScaling=2^0
  Constant : Constant  Value=-2*pi/3  OutDataType=sfix(16)  OutScaling=2^0
  Constant1 : Constant  Value=2*pi/3  OutDataType=sfix(16)  OutScaling=2^0
  Mux1 : Mux  Inputs=[4 4 4]
  Phase A : Subsystem
  Phase B : Subsystem
  Phase C : Subsystem
  Sum : Sum  OutDataType=sfix(16)  OutScaling=2^0  SaturateOnIntegerOverflow=on  InputSameDT=on  OutDataTypeStr=Inherit: Same as first input
  Sum1 : Sum  OutDataType=sfix(16)  OutScaling=2^0  SaturateOnIntegerOverflow=on  InputSameDT=on  OutDataTypeStr=Inherit: Same as first input
  Sum2 : Sum  OutDataType=sfix(16)  OutScaling=2^0  SaturateOnIntegerOverflow=on  InputSameDT=on  OutDataTypeStr=Inherit: Same as first input
  Pulses : Outport  OutDataType=sfix(16)  OutScaling=2^0
  wires:
  Constant1/1 -> Sum1/2
  Sigma/1 -> Phase A/2(sigma), Phase C/2(sigma), Phase B/2(sigma)
  Alpha/1 -> Sum2/2
  wt/1 -> Sum2/1
  Sum2/1 -> Phase A/1(wt), Sum/1, Sum1/1
  Mux1/1 -> Pulses/1
  Phase A/1(Pulses) -> Mux1/1
  Constant/1 -> Sum/2
  Sum/1 -> Phase B/1(wt)
  Sum1/1 -> Phase C/1(wt)
  D_Alpha/1 -> Phase A/3(D_Alpha), Phase B/3(D_Alpha), Phase C/3(D_Alpha)
  Phase B/1(Pulses) -> Mux1/2
  Phase C/1(Pulses) -> Mux1/3

== system with_sssc/sssc Controller/SE Control (UPFC)/Firing Pulses Generator/Bridge 2Y ==
  wt : Inport  PortDimensions=1  OutDataType=sfix(16)  OutScaling=2^0
  Alpha : Inport  Port=2  PortDimensions=1  OutDataType=sfix(16)  OutScaling=2^0
  Sigma : Inport  Port=3  PortDimensions=1  OutDataType=sfix(16)  OutScaling=2^0
  D_Alpha : Inport  Port=4  PortDimensions=1  OutDataType=sfix(16)  OutScaling=2^0
  Constant : Constant  Value=-2*pi/3  OutDataType=sfix(16)  OutScaling=2^0
  Constant1 : Constant  Value=2*pi/3  OutDataType=sfix(16)  OutScaling=2^0
  Mux1 : Mux  Inputs=[4 4 4]
  Phase A : Subsystem
  Phase B : Subsystem
  Phase C : Subsystem
  Sum : Sum  OutDataType=sfix(16)  OutScaling=2^0  SaturateOnIntegerOverflow=on  InputSameDT=on  OutDataTypeStr=Inherit: Same as first input
  Sum1 : Sum  OutDataType=sfix(16)  OutScaling=2^0  SaturateOnIntegerOverflow=on  InputSameDT=on  OutDataTypeStr=Inherit: Same as first input
  Sum2 : Sum  OutDataType=sfix(16)  OutScaling=2^0  SaturateOnIntegerOverflow=on  InputSameDT=on  OutDataTypeStr=Inherit: Same as first input
  Pulses : Outport  OutDataType=sfix(16)  OutScaling=2^0
  wires:
  Phase C/1(Pulses) -> Mux1/3
  Phase B/1(Pulses) -> Mux1/2
  D_Alpha/1 -> Phase C/3(D_Alpha), Phase B/3(D_Alpha), Phase A/3(D_Alpha)
  Sum1/1 -> Phase C/1(wt)
  Sum/1 -> Phase B/1(wt)
  Constant/1 -> Sum/2
  Phase A/1(Pulses) -> Mux1/1
  Mux1/1 -> Pulses/1
  Sum2/1 -> Sum1/1, Sum/1, Phase A/1(wt)
  wt/1 -> Sum2/1
  Alpha/1 -> Sum2/2
  Sigma/1 -> Phase B/2(sigma), Phase C/2(sigma), Phase A/2(sigma)
  Constant1/1 -> Sum1/2

== system with_sssc/sssc Controller/SE Control (UPFC)/Mag/rho and sigma computation/Sigma Computation ==
  note: Mag(pu) = 4 * [ 2/pi * Vdc * sin(sigma/2) ] / [ 500e3*sqrt(2)/sqrt(3) ]
  Mag (pu) : Inport  PortDimensions=1  OutDataType=sfix(16)  OutScaling=2^0
  Vdc (V) : Inport  Port=2  PortDimensions=1  OutDataType=sfix(16)  OutScaling=2^0
  Constant : Constant  Value=0  OutDataType=sfix(16)  OutScaling=2^0
  Constant1 : Constant  Value=1e-6  OutDataType=sfix(16)  OutScaling=2^0
  Constant2 : Constant  Value=pi  OutDataType=sfix(16)  OutScaling=2^0
  Constant3 : Constant  Value=500e3/sqrt(3)*sqrt(2)  OutDataType=sfix(16)  OutScaling=2^0
  Gain : Gain  Gain=2  ParameterDataType=sfix(16)  ParameterScaling=2^0  OutDataType=sfix(16)  OutScaling=2^0  SaturateOnIntegerOverflow=on  OutDataTypeStr=Inherit: Same as input  ParamDataTypeStr=Inherit: Same as input
  Gain2 : Gain  Gain=4*2  ParameterDataType=sfix(16)  ParameterScaling=2^0  OutDataType=sfix(16)  OutScaling=2^0  SaturateOnIntegerOverflow=on  OutDataTypeStr=Inherit: Same as input  ParamDataTypeStr=Inherit: Same as input
  Gain3 : Gain  Gain=180/pi  ParameterDataType=sfix(16)  ParameterScaling=2^0  OutDataType=sfix(16)  OutScaling=2^0  SaturateOnIntegerOverflow=on  OutDataTypeStr=Inherit: Same as input  ParamDataTypeStr=Inherit: Same as input
  Product : Product  Inputs=***/  OutDataType=sfix(16)  OutScaling=2^0  SaturateOnIntegerOverflow=on  InputSameDT=on  OutDataTypeStr=Inherit: Same as first input
  Relational Operator : RelationalOperator  Operator=~=  InputSameDT=on
  Saturation : Saturate  UpperLimit=1  LowerLimit=0  OutDataType=sfix(16)  OutScaling=2^0
  Saturation1 : Saturate  UpperLimit=172.5  LowerLimit=0  OutDataType=sfix(16)  OutScaling=2^0
  Switch1 : Switch  Threshold=0.5  OutDataType=sfix(16)  OutScaling=2^0  SaturateOnIntegerOverflow=on  InputSameDT=on
  Trigonometric Function : Trigonometry  Operator=asin
  sigma (deg) : Outport  OutDataType=sfix(16)  OutScaling=2^0
  wires:
  Saturation1/1 -> sigma (deg)/1
  Gain3/1 -> Saturation1/1
  Gain/1 -> Gain3/1
  Trigonometric Function/1 -> Gain/1
  Saturation/1 -> Trigonometric Function/1
  Constant1/1 -> Switch1/3
  Gain2/1 -> Switch1/1, Relational Operator/1
  Relational Operator/1 -> Switch1/2
  Constant/1 -> Relational Operator/2
  Vdc (V)/1 -> Gain2/1
  Constant3/1 -> Product/3
  Constant2/1 -> Product/2
  Mag (pu)/1 -> Product/1
  Switch1/1 -> Product/4
  Product/1 -> Saturation/1

== system with_sssc/sssc Controller/SE Control (UPFC)/Mag/rho and sigma computation/Vd_Vq--> Mag,rho ==
  Vd_Vq : Inport  PortDimensions=2  OutDataType=sfix(16)  OutScaling=2^0
  Fcn3 : Fcn  Expr=sqrt(u[1]*u[1]+u[2]*u[2])
  Fcn4 : Fcn  Expr=atan2(u[2]+1e-6,u[1])*180/pi
  Mux : Mux  Inputs=2
  Mag_rho : Outport  OutDataType=sfix(16)  OutScaling=2^0
  wires:
  Vd_Vq/1 -> Fcn3/1, Fcn4/1
  Mux/1 -> Mag_rho/1
  Fcn3/1 -> Mux/1
  Fcn4/1 -> Mux/2

== system with_sssc/sssc Controller/SE Control (UPFC)/Measurement System/PQ  Computaion ==
  note: P = Vd*Id + Vq*Iq
  note: Q = Vq*Id-Vd*Iq
  note: PQ Measurement:
  Vd_Vq : Inport  PortDimensions=2  OutDataType=sfix(16)  OutScaling=2^0
  Id_Iq : Inport  Port=2  PortDimensions=2  OutDataType=sfix(16)  OutScaling=2^0
  Demux1 : Demux  Outputs=2
  Demux2 : Demux  Outputs=2
  Mux2 : Mux  Inputs=2
  Product{2..5} (4 alike) : Product  OutDataType=sfix(16)  OutScaling=2^0  SaturateOnIntegerOverflow=on  InputSameDT=on  OutDataTypeStr=Inherit: Same as first input
  Sum : Sum  OutDataType=sfix(16)  OutScaling=2^0  SaturateOnIntegerOverflow=on  InputSameDT=on  OutDataTypeStr=Inherit: Same as first input
  Sum1 : Sum  Inputs=+-  OutDataType=sfix(16)  OutScaling=2^0  SaturateOnIntegerOverflow=on  InputSameDT=on  OutDataTypeStr=Inherit: Same as first input
  P_Q : Outport  OutDataType=sfix(16)  OutScaling=2^0
  wires:
  Product2/1 -> Sum/1
  Product3/1 -> Sum/2
  Product4/1 -> Sum1/1
  Product5/1 -> Sum1/2
  Sum/1 -> Mux2/1
  Sum1/1 -> Mux2/2
  Mux2/1 -> P_Q/1
  Vd_Vq/1 -> Demux1/1
  Id_Iq/1 -> Demux2/1
  Demux1/2 -> Product3/1, Product4/1
  Demux2/1 -> Product2/2, Product4/2
  Demux1/1 -> Product2/1, Product5/1
  Demux2/2 -> Product3/2, Product5/2

== system with_sssc/sssc Controller/SE Control (UPFC)/Measurement System/Voltage Measurement ==
  note: Pierre Giroux, Gilbert Sybille
      | Power System Simulation Laboratory
      | IREQ, Hydro-Quebc
  note: Discrete 3-phase PLL-Driven Positive-Sequence Fundamental Value
  Freq : Inport  OutDataType=sfix(16)  OutScaling=2^0
  Sin_Cos : Inport  Port=2  PortDimensions=2  OutDataType=sfix(16)  OutScaling=2^0
  abc : Inport  Port=3  PortDimensions=3  OutDataType=sfix(16)  OutScaling=2^0
  Demux : Demux  Outputs=3
  Discrete Variable Frequency Mean value1 : Subsystem  mask(Discrete Variable-Frequency Mean Value){Finit=Finit, Vinit=Real_Init, Ts=Ts}
      mask prompts: Finit "Initial Frequency (Hz):"; Vinit "Initial input (DC component):"; Ts "Sample time:"
      mask help:
      | This discrete block computes the mean value of the input signal (port In) over a running window of one cycle of a specified frequency (port Freq).
      |
      | For the first cycle of simulation (specified by the parameter "Initial frequency"), the output is held to the value of the  "Initial input" parameter.
  Discrete Variable Frequency Mean value2 : Subsystem  mask(Discrete Variable-Frequency Mean Value){Finit=Finit, Vinit=Imag_Init, Ts=Ts}
      mask prompts: Finit "Initial Frequency (Hz):"; Vinit "Initial input (DC component):"; Ts "Sample time:"
      mask help:
      | This discrete block computes the mean value of the input signal (port In) over a running window of one cycle of a specified frequency (port Freq).
      |
      | For the first cycle of simulation (specified by the parameter "Initial frequency"), the output is held to the value of the  "Initial input" parameter.
  Mux1 : Mux  Inputs=2
  Terminator : Terminator
  abc_to_dq0 Transformation : powerlib_extras/Measurements/abc_to_dq0 Transformation  DialogController=POWERSYS.PowerSysDialog  SystemSampleTime=-1
  VdVq : Outport  OutDataType=sfix(16)  OutScaling=2^0
  wires:
  Discrete Variable Frequency Mean value1/1(Mean) -> Mux1/1  "Real"
  Discrete Variable Frequency Mean value2/1(Mean) -> Mux1/2  "Imag"
  Sin_Cos/1 -> abc_to_dq0 Transformation/2
  Freq/1 -> Discrete Variable Frequency Mean value2/1(Freq), Discrete Variable Frequency Mean value1/1(Freq)
  Demux/2 -> Discrete Variable Frequency Mean value2/2(In)
  Demux/1 -> Discrete Variable Frequency Mean value1/2(In)
  abc/1 -> abc_to_dq0 Transformation/1
  abc_to_dq0 Transformation/1 -> Demux/1
  Demux/3 -> Terminator/1
  Mux1/1 -> VdVq/1

== system with_sssc/sssc Controller/SE Control (UPFC)/Measurement System/Voltage Measurement1 ==
  note: Discrete 3-phase PLL-Driven Positive-Sequence Fundamental Value
  note: Pierre Giroux, Gilbert Sybille
      | Power System Simulation Laboratory
      | IREQ, Hydro-Quebc
  Freq : Inport  OutDataType=sfix(16)  OutScaling=2^0
  Sin_Cos : Inport  Port=2  PortDimensions=2  OutDataType=sfix(16)  OutScaling=2^0
  abc : Inport  Port=3  PortDimensions=3  OutDataType=sfix(16)  OutScaling=2^0
  Demux : Demux  Outputs=3
  Discrete Variable Frequency Mean value1 : Subsystem  mask(Discrete Variable-Frequency Mean Value){Finit=Finit, Vinit=Real_Init, Ts=Ts}
      mask prompts: Finit "Initial Frequency (Hz):"; Vinit "Initial input (DC component):"; Ts "Sample time:"
      mask help:
      | This discrete block computes the mean value of the input signal (port In) over a running window of one cycle of a specified frequency (port Freq).
      |
      | For the first cycle of simulation (specified by the parameter "Initial frequency"), the output is held to the value of the  "Initial input" parameter.
  Discrete Variable Frequency Mean value2 : Subsystem  mask(Discrete Variable-Frequency Mean Value){Finit=Finit, Vinit=Imag_Init, Ts=Ts}
      mask prompts: Finit "Initial Frequency (Hz):"; Vinit "Initial input (DC component):"; Ts "Sample time:"
      mask help:
      | This discrete block computes the mean value of the input signal (port In) over a running window of one cycle of a specified frequency (port Freq).
      |
      | For the first cycle of simulation (specified by the parameter "Initial frequency"), the output is held to the value of the  "Initial input" parameter.
  Mux1 : Mux  Inputs=2
  Terminator : Terminator
  abc_to_dq0 Transformation : powerlib_extras/Measurements/abc_to_dq0 Transformation  DialogController=POWERSYS.PowerSysDialog  SystemSampleTime=-1
  IdIq : Outport  OutDataType=sfix(16)  OutScaling=2^0
  wires:
  Mux1/1 -> IdIq/1
  Demux/3 -> Terminator/1
  abc_to_dq0 Transformation/1 -> Demux/1
  abc/1 -> abc_to_dq0 Transformation/1
  Demux/1 -> Discrete Variable Frequency Mean value1/2(In)
  Demux/2 -> Discrete Variable Frequency Mean value2/2(In)
  Freq/1 -> Discrete Variable Frequency Mean value1/1(Freq), Discrete Variable Frequency Mean value2/1(Freq)
  Sin_Cos/1 -> abc_to_dq0 Transformation/2
  Discrete Variable Frequency Mean value2/1(Mean) -> Mux1/2  "Imag"
  Discrete Variable Frequency Mean value1/1(Mean) -> Mux1/1  "Real"

== system with_sssc/sssc Controller/SE Control (UPFC)/Vd,Vq Selection (Auto/Man) and Limit Computation/Vd,Vq Selection and Limit Computation ==
  Vd_Vq(auto)* : Inport  PortDimensions=2  OutDataType=sfix(16)  OutScaling=2^0
  OpMode : Inport  Port=2  PortDimensions=1  OutDataType=sfix(16)  OutScaling=2^0
  Mag* (man) : Inport  Port=3  PortDimensions=1  OutDataType=sfix(16)  OutScaling=2^0
  rho* (man) : Inport  Port=4  PortDimensions=1  OutDataType=sfix(16)  OutScaling=2^0
  Mux : Mux  Inputs=2
  Product : Product  OutDataType=sfix(16)  OutScaling=2^0  SaturateOnIntegerOverflow=on  InputSameDT=on  OutDataTypeStr=Inherit: Same as first input
  Rate Limiter 3 : powerlib_extras/Discrete  Control Blocks/Discrete Rate Limiter  DialogController=POWERSYS.PowerSysDialog  SystemSampleTime=-1  R=0.025*60  F=-0.025*60  Vinit=0  Ts=Ts
  Switch : Switch  Threshold=0.5  OutDataType=sfix(16)  OutScaling=2^0  SaturateOnIntegerOverflow=on  InputSameDT=on
  Trigonometric Function : Trigonometry
  Trigonometric Function1 : Trigonometry  Operator=cos
  Vd,Vq Limit  Computation : Subsystem
  deg->rad : Gain  Gain=pi/180  ParameterDataType=sfix(16)  ParameterScaling=2^0  OutDataType=sfix(16)  OutScaling=2^0  SaturateOnIntegerOverflow=on  OutDataTypeStr=Inherit: Same as input  ParamDataTypeStr=Inherit: Same as input
  VdVq : Outport  OutDataType=sfix(16)  OutScaling=2^0
  wires:
  OpMode/1 -> Switch/2
  Trigonometric Function1/1 -> Mux/1
  Trigonometric Function/1 -> Mux/2
  Mux/1 -> Product/2
  rho* (man)/1 -> deg->rad/1
  Mag* (man)/1 -> Product/1
  deg->rad/1 -> Trigonometric Function1/1, Trigonometric Function/1
  Switch/1 -> Vd,Vq Limit  Computation/1(VdVq*)  "VdVq*"
  Product/1 -> Rate Limiter 3/1
  Vd,Vq Limit  Computation/1(VdVq) -> VdVq/1
  Vd_Vq(auto)*/1 -> Switch/3
  Rate Limiter 3/1 -> Switch/1

== system with_sssc/sssc Controller/SH Control (STATCOM)/DC Balance Regulator/ Mean value ==
  note: Pierre Giroux, Gilbert Sybille
      | Power System Simulation Laboratory
      | IREQ, Hydro-Quebc
  note: Discrete Mean Value
  In : Inport  OutDataType=sfix(16)  OutScaling=2^0
  Constant : Constant  Value=Vinit  OutDataType=sfix(16)  OutScaling=2^0
  Constant1 : Constant  Value=Correction  OutDataType=sfix(16)  OutScaling=2^0
  Integ4 : DiscreteIntegrator  IntegratorMethod=Integration: Trapezoidal  SampleTime=Ts  OutDataType=sfix(16)  OutScaling=2^0  ICPrevOutput=DiscIntNeverNeededParam  ICPrevScaledInput=DiscIntNeverNeededParam
  K2 : Constant  Value=Freq  OutDataType=sfix(16)  OutScaling=2^0
  Product : Product  OutDataType=sfix(16)  OutScaling=2^0  SaturateOnIntegerOverflow=on  InputSameDT=on  OutDataTypeStr=Inherit: Same as first input
  Product1 : Product  Inputs=**  OutDataType=sfix(16)  OutScaling=2^0  SaturateOnIntegerOverflow=on  InputSameDT=on  OutDataTypeStr=Inherit: Same as first input
  Step : Step  Time=1/Freq  SampleTime=Ts
  Sum5 : Sum  OutDataType=sfix(16)  OutScaling=2^0  SaturateOnIntegerOverflow=on  InputSameDT=on  OutDataTypeStr=Inherit: Same as first input
  Sum7 : Sum  Inputs=-+  OutDataType=sfix(16)  OutScaling=2^0  SaturateOnIntegerOverflow=on  InputSameDT=on  OutDataTypeStr=Inherit: Same as first input
  Switch : Switch  Threshold=0.5  OutDataType=sfix(16)  OutScaling=2^0  SaturateOnIntegerOverflow=on  InputSameDT=on
  Transport Delay : TransportDelay  DelayTime=Delay
  Mean : Outport  OutDataType=sfix(16)  OutScaling=2^0
  wires:
  Product/1 -> Sum5/1  "Mean value"
  Transport Delay/1 -> Sum7/1
  Sum7/1 -> Product/1
  Integ4/1 -> Transport Delay/1, Sum7/2
  K2/1 -> Product/2
  In/1 -> Integ4/1, Product1/1  "In"
  Constant1/1 -> Product1/2
  Product1/1 -> Sum5/2  "Correction"
  Sum5/1 -> Switch/1
  Step/1 -> Switch/2
  Constant/1 -> Switch/3
  Switch/1 -> Mean/1

== system with_sssc/sssc Controller/SH Control (STATCOM)/DC Balance Regulator/PI Regulator ==
  note: Pierre Giroux, Gilbert Sybille
      | Power System Simulation Laboratory
      | IREQ, Hydro-Quebc
  note: Discrete PID Controller
  Error : Inport  OutDataType=sfix(16)  OutScaling=2^0
  Reset : Inport  Port=2  OutDataType=sfix(16)  OutScaling=2^0
  Discrete-Time Integrator : DiscreteIntegrator  ExternalReset=rising  InitialCondition=Init  SampleTime=Ts  OutDataType=sfix(16)  OutScaling=2^0  LimitOutput=on  UpperSaturationLimit=UpperLimit  LowerSaturationLimit=LowerLimit  ICPrevOutput=DiscIntNeverNeededParam  ICPrevScaledInput=DiscIntNeverNeededParam
  Kp4 : Gain  Gain=Kp  ParameterDataType=sfix(16)  ParameterScaling=2^0  OutDataType=sfix(16)  OutScaling=2^0  SaturateOnIntegerOverflow=on  OutDataTypeStr=Inherit: Same as input  ParamDataTypeStr=Inherit: Same as input
  Kp5 : Gain  Gain=Ki  ParameterDataType=sfix(16)  ParameterScaling=2^0  OutDataType=sfix(16)  OutScaling=2^0  SaturateOnIntegerOverflow=on  OutDataTypeStr=Inherit: Same as input  ParamDataTypeStr=Inherit: Same as input
  Saturation2 : Saturate  UpperLimit=UpperLimit  LowerLimit=LowerLimit  OutDataType=sfix(16)  OutScaling=2^0
  Sum6 : Sum  OutDataType=sfix(16)  OutScaling=2^0  SaturateOnIntegerOverflow=on  InputSameDT=on  OutDataTypeStr=Inherit: Same as first input
  Out : Outport  OutDataType=sfix(16)  OutScaling=2^0  InitialOutput=0
  wires:
  Saturation2/1 -> Out/1
  Discrete-Time Integrator/1 -> Sum6/2
  Kp4/1 -> Sum6/1
  Kp5/1 -> Discrete-Time Integrator/1
  Sum6/1 -> Saturation2/1
  Error/1 -> Kp5/1, Kp4/1
  Reset/1 -> Discrete-Time Integrator/2

== system with_sssc/sssc Controller/SH Control (STATCOM)/Firing Pulses Generator/Bridge 1D ==
  wt : Inport  PortDimensions=1  OutDataType=sfix(16)  OutScaling=2^0
  Alpha : Inport  Port=2  PortDimensions=1  OutDataType=sfix(16)  OutScaling=2^0
  Sigma : Inport  Port=3  PortDimensions=1  OutDataType=sfix(16)  OutScaling=2^0
  D_Alpha : Inport  Port=4  PortDimensions=1  OutDataType=sfix(16)  OutScaling=2^0
  Constant : Constant  Value=-2*pi/3  OutDataType=sfix(16)  OutScaling=2^0
  Constant1 : Constant  Value=2*pi/3  OutDataType=sfix(16)  OutScaling=2^0
  Mux1 : Mux  Inputs=[4 4 4]
  Phase A : Subsystem
  Phase B : Subsystem
  Phase C : Subsystem
  Sum : Sum  OutDataType=sfix(16)  OutScaling=2^0  SaturateOnIntegerOverflow=on  InputSameDT=on  OutDataTypeStr=Inherit: Same as first input
  Sum1 : Sum  OutDataType=sfix(16)  OutScaling=2^0  SaturateOnIntegerOverflow=on  InputSameDT=on  OutDataTypeStr=Inherit: Same as first input
  Sum2 : Sum  OutDataType=sfix(16)  OutScaling=2^0  SaturateOnIntegerOverflow=on  InputSameDT=on  OutDataTypeStr=Inherit: Same as first input
  Pulses : Outport  OutDataType=sfix(16)  OutScaling=2^0
  wires:
  Constant1/1 -> Sum1/2
  Sigma/1 -> Phase A/2(sigma), Phase C/2(sigma), Phase B/2(sigma)
  Alpha/1 -> Sum2/2
  wt/1 -> Sum2/1
  Sum2/1 -> Phase A/1(wt), Sum/1, Sum1/1
  Mux1/1 -> Pulses/1
  Phase A/1(Pulses) -> Mux1/1
  Constant/1 -> Sum/2
  Sum/1 -> Phase B/1(wt)
  Sum1/1 -> Phase C/1(wt)
  D_Alpha/1 -> Phase A/3(D_Alpha), Phase B/3(D_Alpha), Phase C/3(D_Alpha)
  Phase B/1(Pulses) -> Mux1/2
  Phase C/1(Pulses) -> Mux1/3
